simulink model "bchdect2"  (Simulink 7.2)
settings: Solver=ode45  StartTime=0.0  StopTime=10.0  RelTol=1e-3
undefined symbols (not defined in the file or in its folder): dvbkBCH
libraries: commblkcod2 x1
settings Model: Creator=sayazgok  LastModifiedBy=sayazgok

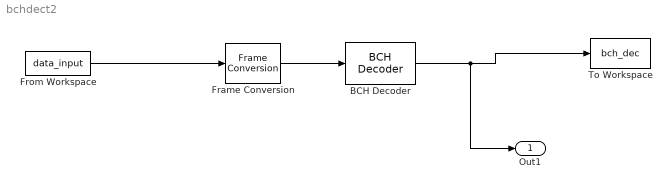
== system bchdect2 ==
  BCH Decoder : commblkcod2/BCH Decoder  n=dvbnBCH  k=dvbkBCH  specPrimPoly=on  prPoly=dvbprimBCH  specGenPoly=on  genPoly=dvbgenBCH  specDisableGenCheck=on  specPuncture=off  punctVec=[ones(8,1); zeros(2,1)]  specErasurePort=off  showNumErr=off
  Frame Conversion : FrameConversion
  From Workspace : FromWorkspace  VariableName=data_input  SampleTime=0
  To Workspace : ToWorkspace  VariableName=bch_dec  SampleTime=-1  SaveFormat=Array
  Out1 : Outport  OutDataType=sfix(16)  OutScaling=2^0
  wires:
  Frame Conversion/1 -> BCH Decoder/1
  From Workspace/1 -> Frame Conversion/1
  BCH Decoder/1 -> To Workspace/1, Out1/1
